simulink library "Analog"  (R2017a)
settings: Solver=VariableStepAuto  StartTime=0.0  StopTime=10.0  RelTol=1e-3
settings Model: Creator=Di Russo  LastModifiedBy=Vraj M

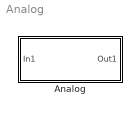
== system Analog ==
  Analog : Subsystem

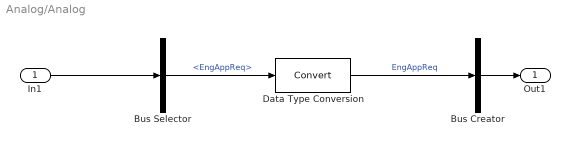
== system Analog/Analog ==
  In1 : Inport
  Bus Creator : BusCreator  Inputs=1
  Bus Selector : BusSelector  OutputSignals=Controls.EngAppReq
  Data Type Conversion : DataTypeConversion
  Out1 : Outport
  wires:
  Data Type Conversion/1 -> Bus Creator/1  "EngAppReq"
  Bus Selector/1 -> Data Type Conversion/1  "<EngAppReq>"
  Bus Creator/1 -> Out1/1
  In1/1 -> Bus Selector/1
